simulink model "distance_model"  (R2016b)
settings: Solver=VariableStepAuto  StartTime=0.0  StopTime=10.0  RelTol=1e-3
settings Model: Creator=202008840  LastModifiedBy=202008840

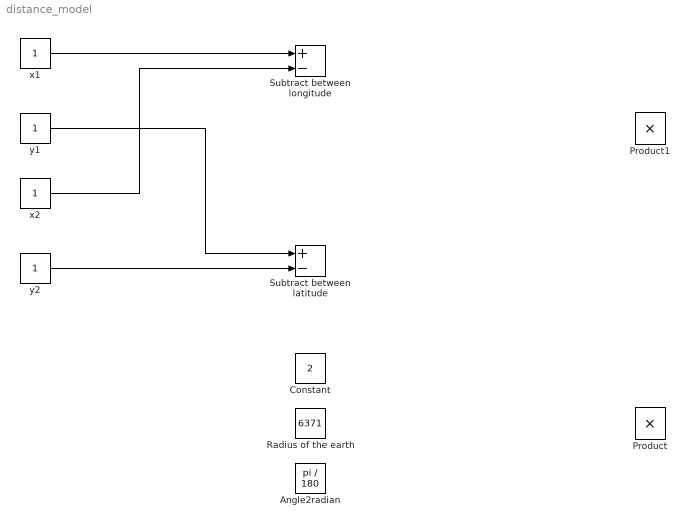
== system distance_model ==
  Angle2radian : Constant  Value=pi / 180
  Constant : Constant  Value=2
  Product : Product  Inputs=4
  Product1 : Product  Inputs=3
  Radius of the earth : Constant  Value=6371
  Subtract between latitude : Sum  Inputs=+-
  Subtract between longitude : Sum  Inputs=+-
  x1 : Constant
  x2 : Constant
  y1 : Constant
  y2 : Constant
  wires:
  x1/1 -> Subtract between longitude/1
  x2/1 -> Subtract between longitude/2
  y1/1 -> Subtract between latitude/1
  y2/1 -> Subtract between latitude/2
